simulink model "ev"  (R2021a)
settings: Solver=ode4  StartTime=0  StopTime=1082  FixedStep=sim_dt  RelTol=1e-3
model workspace (MAT data in the model file):
  T_eff_bp = [-270; -210; -150; -90; -30; 30; 90; 150; 210; 270]
  T_eff_bp_2 = [-270; -210; -150; -90; -30; 30; 90; 150; 210; 270]
  losses_table = [108927.107777 7820.2782368 7820.17609997 7820.2782368 7820.2782368 7820.2782368 7820.2782368 7820.26172359 7820.2782368 9345.38006027 108927.107777 7820.2782368 ... (100 elements, 10x10)]
  losses_table_2 = [108927.107777 7820.2782368 7820.17609997 7820.2782368 7820.2782368 7820.2782368 7820.2782368 7820.26172359 7820.2782368 9345.38006027 108927.107777 7820.2782368 ... (100 elements, 10x10)]
  w_eff_bp = [0; 888.888888889; 1777.77777778; 2666.66666667; 3555.55555556; 4444.44444444; 5333.33333333; 6222.22222222; 7111.11111111; 8000]
  w_eff_bp_2 = [0; 888.888888889; 1777.77777778; 2666.66666667; 3555.55555556; 4444.44444444; 5333.33333333; 6222.22222222; 7111.11111111; 8000]
undefined symbols (not defined in the file): Af, alpha, Bt, C, C_fa, C_free, C_sa_bat, C_sa_uc, Cd, Cmax, Continuous, Crr, DoD, effi, etaFD, etaG, FD, G, gear, Iucmax, m, M1m, M2m, Max, npar, npar_free, npara, nparf, nparfa, nparsa_bat, nparsa_UC, nser, nser_free, nserfa, nsersa_bat, nsersa_UC, Qbat, regenmax, Ri_BP, RL, ro, Rsc, Rsc_A, Rsc_F, Rsc_sa_bat, Rsc_sa_uc, rw, sim_dt, SOC_BP, SoCbatmax, SoCbatmin, SoCucmax, SoCucmin, speed, torque, VinBat, Voc_BP, Vuc, Vuc_fa, Vuc_free ... (+2)
libraries: autolibshared x41, simulink x26, autolibdcdc x13, autolibdatasheetbattery x7, autolibmappedmotor x6, fl_lib x3, nesl_utility x3, spsSupercapacitorLib x3, pid_lib x1
(part 5 of 18)

== system ev/Tesis/battery model limitedmod ==
  motor_pwr_contr : Inport
  Gain : Gain  Gain=nser
  Gain1 : Gain  Gain=nser/npar
  Gain11 : Gain  Gain=(Qbat*VinBat*nser*npar)
  Gain2 : Gain  Gain=1/(Qbat*VinBat*nser*npar*3600)
  Gain3 : Gain  Gain=-1
  Ibatt1 : Scope
  Integrator2 : Integrator
  MATLAB Function : MATLAB Function  TreatAsAtomicUnit=on
  MATLAB Function2 : MATLAB Function  TreatAsAtomicUnit=on
  Mux13 : Mux  Inputs=3
  Mux14 : Mux  Inputs=3
  OCV : Lookup_n-D  NumberOfTableDimensions=1  BreakpointsForDimension1=SOC_BP  Table=Voc_BP  InternalRulePriority=Speed  RndMeth=Simplest  InputSameDT=on
  PMG_max : Lookup_n-D  NumberOfTableDimensions=1  BreakpointsForDimension1=SOC_BP  Table=Voc_BP*nser*1*50*npar  InternalRulePriority=Speed  RndMeth=Simplest  InputSameDT=on
  PMG_min : Lookup_n-D  NumberOfTableDimensions=1  BreakpointsForDimension1=SOC_BP  Table=-Voc_BP*nser*1*50*npar  InternalRulePriority=Speed  RndMeth=Simplest  InputSameDT=on
  Polim : Scope
  Pow1 : Scope
  Product : Product
  Product1 : Product
  Ri : Lookup_n-D  NumberOfTableDimensions=1  BreakpointsForDimension1=SOC_BP  Table=Ri_BP  InternalRulePriority=Speed  RndMeth=Simplest  InputSameDT=on
  Ri4 : Lookup_n-D  NumberOfTableDimensions=1  BreakpointsForDimension1=SOC_BP  Table=Ri_BP  InternalRulePriority=Speed  RndMeth=Simplest  InputSameDT=on
  SOC : Integrator  InitialCondition=(1-DoD)
  Saturation Dynamic : simulink/Discontinuities/Saturation Dynamic  OutMin=[]  OutMax=[]  OutDataTypeStr=Inherit: Same as second input  OutDataType=fixdt(1, 16)  OutScaling=2^-10  DoSatur=off
  Scope42 : Scope
  Scope43 : Scope
  Scope45 : Scope
  SoC : Scope  NumInputPorts=2
  Subtract : Sum  Inputs=+-
  Switch13 : Switch  Criteria=u2 > Threshold
  Vo : Scope
  Voc : Scope
  ener Wh : Scope
  iR : Scope
  iRt : Scope
  tag scope: modi=global
  wires:
  Mux13/1 -> Scope42/1
  PMG_min/1 -> Saturation Dynamic/3, Scope43/1, Mux13/3
  Switch13/1 -> Gain1/1, iR/1
  Gain/1 -> MATLAB Function/1(OCV), Subtract/1, Mux14/2, Voc/1  "OCV"
  Gain11/1 -> ener Wh/1
  Gain2/1 -> Integrator2/1, SOC/1
  motor_pwr_contr/1 -> Saturation Dynamic/2, Switch13/2, Mux13/1, MATLAB Function2/3(Pmot)
  Saturation Dynamic/1 -> Polim/1, MATLAB Function/3(P)
  Gain1/1 -> MATLAB Function2/1(Ri), Product1/2, MATLAB Function/2(Ri), iRt/1
  Ri/1 -> Switch13/1
  Ri4/1 -> Switch13/3
  MATLAB Function/1(I_batt) -> Ibatt1/1, Product1/1, MATLAB Function2/2(Ib), Product/2
  OCV/1 -> Vo/1, Gain/1
  Mux14/1 -> Scope45/1
  SOC/1 -> [modi], PMG_max/1, PMG_min/1, OCV/1, Ri/1, Ri4/1, SoC/1  "SOC"
  PMG_max/1 -> Saturation Dynamic/1, Mux13/2
  Integrator2/1 -> Gain11/1
  MATLAB Function2/1(Vb) -> Mux14/1  "Vb"
  Product/1 -> Pow1/1, Gain3/1, Gain2/1
  Product1/1 -> Subtract/2
  Subtract/1 -> Product/1, Mux14/3

== system ev/Drive cycle power demand/Veh force estimation/Aerodynamic_drag ==
  vel_m/s : Inport
  air_density : Inport  Port=2
  frontal_area : Inport  Port=3
  Drag_coefficient : Inport  Port=4
  Constant : Constant  Value=0.5
  Math Function : Math  Operator=square  SignedPower=on  SaturateOnIntegerOverflow=on
  Product : Product  Inputs=5
  Fad : Outport  VectorParamsAs1DForOutWhenUnconnected=off
  wires:
  Product/1 -> Fad/1  "Aerodynamic_drag"
  Math Function/1 -> Product/4
  vel_m/s/1 -> Math Function/1
  Constant/1 -> Product/5
  air_density/1 -> Product/1
  frontal_area/1 -> Product/2
  Drag_coefficient/1 -> Product/3

== system ev/Drive cycle power demand/Veh force estimation/Hill_climbing_force ==
  vel_m/s : Inport
  vehicle_mass : Inport  Port=2
  Gravity : Inport  Port=3
  Theta : Inport  Port=4
  Constant : Constant  Value=0
  Divide : Product  Inputs=*/
  Gain : Gain  Gain=pi/180
  Product : Product  Inputs=4
  Switch : Switch  Criteria=u2 ~= 0
  Trigonometric Function : Trigonometry
  Fhc : Outport  VectorParamsAs1DForOutWhenUnconnected=off
  wires:
  Product/1 -> Fhc/1
  vehicle_mass/1 -> Product/2
  Theta/1 -> Gain/1
  Gravity/1 -> Product/3
  Trigonometric Function/1 -> Product/4
  Gain/1 -> Trigonometric Function/1
  Constant/1 -> Switch/3
  Switch/1 -> Product/1
  Divide/1 -> Switch/1
  vel_m/s/1 -> Divide/1, Divide/2, Switch/2

== system ev/Drive cycle power demand/Veh force estimation/Linear_acceleration ==
  Acceleration : Inport
  Veh_mass : Inport  Port=2
  Constant : Constant  Value=1.05
  Product : Product  Inputs=3
  Fhc : Outport  VectorParamsAs1DForOutWhenUnconnected=off
  wires:
  Product/1 -> Fhc/1
  Acceleration/1 -> Product/1
  Constant/1 -> Product/3
  Veh_mass/1 -> Product/2

== system ev/Drive cycle power demand/Veh force estimation/Rolling resistance ==
  vehicle_mass : Inport
  Rolling_resistance : Inport  Port=2
  gravity : Inport  Port=3
  theta : Inport  Port=4
  v m/s : Inport  Port=5
  Gain : Gain  Gain=pi/180
  Interpreted MATLAB Function : MATLABFcn  MATLABFcn=sign
  Product : Product  Inputs=4
  Product1 : Product
  Scope : Scope
  Trigonometric Function : Trigonometry  Operator=cos
  Fhc : Outport  VectorParamsAs1DForOutWhenUnconnected=off
  wires:
  vehicle_mass/1 -> Product/1
  gravity/1 -> Product/3
  Rolling_resistance/1 -> Product/2
  v m/s/1 -> Interpreted MATLAB Function/1
  Product/1 -> Product1/1
  Product1/1 -> Fhc/1
  Interpreted MATLAB Function/1 -> Product1/2, Scope/1
  Trigonometric Function/1 -> Product/4
  Gain/1 -> Trigonometric Function/1
  theta/1 -> Gain/1

== system ev/Tesis/Battery model/Subsystem ==
  power : Inport
  motor_pwr_contr : Inport  Port=2
  1-D Lookup Table : Lookup_n-D  NumberOfTableDimensions=1  BreakpointsForDimension1=Continuous(:,1)  Table=Continuous(:,2)  InternalRulePriority=Speed  RndMeth=Simplest  InputSameDT=on
  1-D Lookup Table2 : Lookup_n-D  NumberOfTableDimensions=1  BreakpointsForDimension1=Continuous(:,1)  Table=-Continuous(:,2)  InternalRulePriority=Speed  RndMeth=Simplest  InputSameDT=on
  Constant : Constant  Value=0
  Constant1 : Constant
  Divide1 : Product  Inputs=**
  Divide2 : Product  Inputs=**
  Divide3 : Product  Inputs=*/
  Gain2 : Gain  Gain=30/pi
  Gain4 : Gain  Gain=0.95
  Gain5 : Gain  Gain=1/rw
  Gain6 : Gain  Gain=1/0.95
  Manual Switch : ManualSwitch  CurrentSetting=0
  Saturation Dynamic : simulink/Discontinuities/Saturation Dynamic  OutMin=[]  OutMax=[]  OutDataTypeStr=Inherit: Same as second input  OutDataType=fixdt(1, 16)  OutScaling=2^-10  DoSatur=off
  Scope : Scope
  Scope1 : Scope
  Switch : Switch  Criteria=u2 ~= 0
  Switch1 : Switch
  Switch2 : Switch  Criteria=u2 ~= 0
  motor speed estimation : Subsystem
  Out1 : Outport
  wires:
  motor_pwr_contr/1 -> Switch1/2
  Gain4/1 -> Divide1/1  "breaking torque"
  [gear_ratio] -> Divide1/2
  Divide1/1 -> Switch1/1
  Switch1/1 -> Gain5/1  "motor torque"
  Gain5/1 -> Out1/1  "FORCE"
  [gear_ratio] -> Divide2/2
  Gain6/1 -> Divide2/1  "motor_torque"
  Divide2/1 -> Switch1/3
  Divide3/1 -> Switch/1, Scope/1  "torque"
  power/1 -> Divide3/1  "power"
  Gain2/1 -> 1-D Lookup Table2/1, 1-D Lookup Table/1
  1-D Lookup Table/1 -> Saturation Dynamic/1
  1-D Lookup Table2/1 -> Saturation Dynamic/3
  Saturation Dynamic/1 -> Gain4/1, Gain6/1
  Switch/1 -> Saturation Dynamic/2
  Constant/1 -> Switch/3
  motor speed estimation/1(motor angular speed) -> Manual Switch/2  "motor angular speed required"
  Manual Switch/1 -> Scope1/1, Gain2/1, Switch2/1, Switch2/2, Switch/2
  [mtr_speed] -> Manual Switch/1
  [Veh_real_bat1] -> motor speed estimation/1(vel_m/s)
  Switch2/1 -> Divide3/2
  Constant1/1 -> Switch2/3
